simulink model "Logic_Gates"  (R2021a)
settings: Solver=VariableStepAuto  StartTime=0.0  StopTime=10.0  RelTol=1e-3
settings Model: Creator=isacperez  LastModifiedBy=isacperez

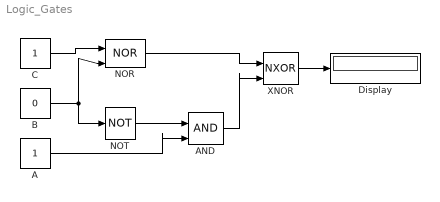
== system Logic_Gates ==
  A : Constant
  AND : Logic  IconShape=distinctive  AllPortsSameDT=off  OutDataTypeStr=boolean
  B : Constant  Value=0
  C : Constant
  Display : Display
  NOR : Logic  Operator=NOR  IconShape=distinctive  AllPortsSameDT=off  OutDataTypeStr=boolean
  NOT : Logic  Operator=NOT  IconShape=distinctive  AllPortsSameDT=off  OutDataTypeStr=boolean
  XNOR : Logic  Operator=NXOR  IconShape=distinctive  AllPortsSameDT=off  OutDataTypeStr=boolean
  wires:
  C/1 -> NOR/1
  B/1 -> NOT/1, NOR/2
  NOT/1 -> AND/1
  A/1 -> AND/2
  AND/1 -> XNOR/2
  NOR/1 -> XNOR/1
  XNOR/1 -> Display/1
